simulink model "simple_echo"  (R2019a)
settings: Solver=VariableStepAuto  StartTime=0.0  StopTime=10.0  RelTol=1e-3
settings Model: Creator=amyel  LastModifiedBy=h34j161

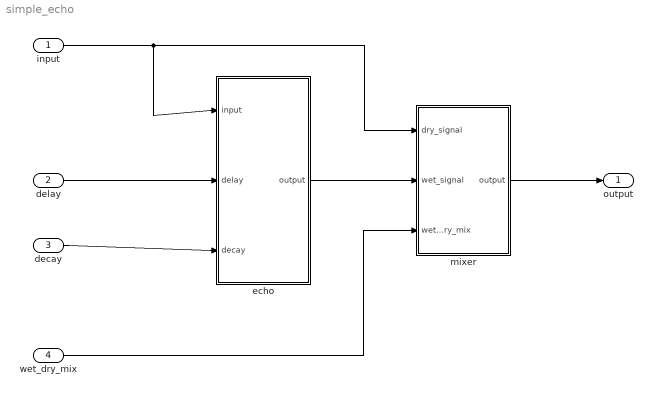
== system simple_echo ==
  input : Inport
  delay : Inport  Port=2
  decay : Inport  Port=3
  wet_dry_mix : Inport  Port=4
  echo : Subsystem
  mixer : Subsystem
  output : Outport
  wires:
  echo/1(output) -> mixer/2(wet_signal)
  wet_dry_mix/1 -> mixer/3(wet_dry_mix)
  input/1 -> echo/1(input), mixer/1(dry_signal)
  mixer/1(output) -> output/1
  decay/1 -> echo/3(decay)
  delay/1 -> echo/2(delay)

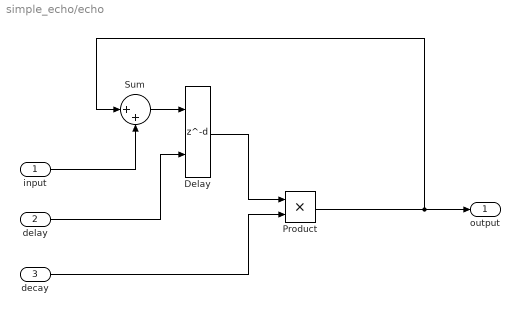
== system simple_echo/echo ==
  input : Inport
  delay : Inport  Port=2
  decay : Inport  Port=3
  Delay : Delay  DelayLengthSource=Input port  DelayLengthUpperLimit=Fs  DiagnosticForDelayLength=Error  UseCircularBuffer=on
      settings: InputPortMap=u0,p1
  Product : Product
  Sum : Sum  Inputs=|++
  output : Outport
  wires:
  delay/1 -> Delay/2
  Product/1 -> Sum/1, output/1
  decay/1 -> Product/2
  Delay/1 -> Product/1
  input/1 -> Sum/2
  Sum/1 -> Delay/1

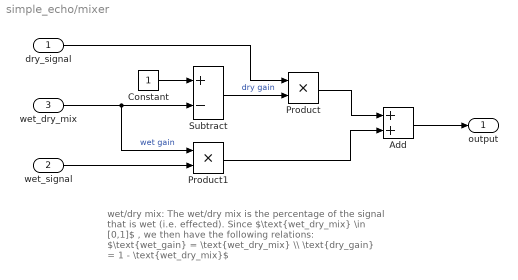
== system simple_echo/mixer ==
  note: wet/dry mix:
      | The wet/dry mix is the percentage of the signal that is wet (i.e. effected).
      |
      | Since $\text{wet_dry_mix} \in [0,1]$ , we then have the following relations:
      | $\text{wet_gain} = \text{wet_dry_mix} \\ \text{dry_gain} = 1 - \text{wet_dry_mix}$
  dry_signal : Inport
  wet_signal : Inport  Port=2
  wet_dry_mix : Inport  Port=3
  Add : Sum
  Constant : Constant  SampleTime=-1
  Product : Product
  Product1 : Product
  Subtract : Sum  Inputs=+-
  output : Outport
  wires:
  Add/1 -> output/1
  Constant/1 -> Subtract/1
  wet_dry_mix/1 -> Product1/1, Subtract/2  "wet gain"
  Product/1 -> Add/1
  Product1/1 -> Add/2
  wet_signal/1 -> Product1/2
  dry_signal/1 -> Product/1
  Subtract/1 -> Product/2  "dry gain"
